simulink model "Comunicacion_taller"  (R2023a)
settings: Solver=VariableStepAuto  StartTime=0.0  StopTime=5  RelTol=1e-3
libraries: instrumentseriallib x2
settings Model: Creator=Sergio  LastModifiedBy=santi
settings DebuggingCC: UnconnectedInputMsg=warning  UnconnectedOutputMsg=warning  UnconnectedLineMsg=warning
settings ModelReferenceCC: EnableRefExpFcnMdlSchedulingChecks=on
settings RTWCC: DLArmComputeVersion=19.05

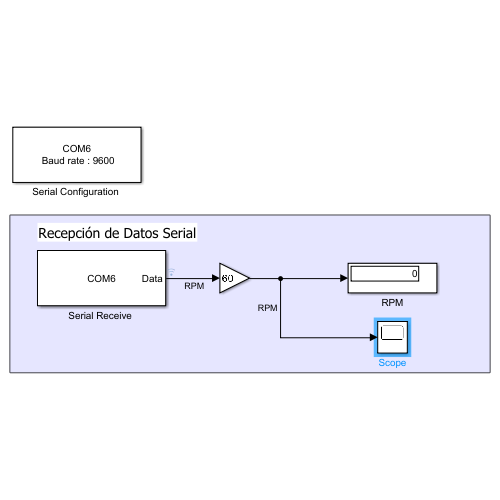
[thumbnail: Simulink's stored preview of the top-level diagram]
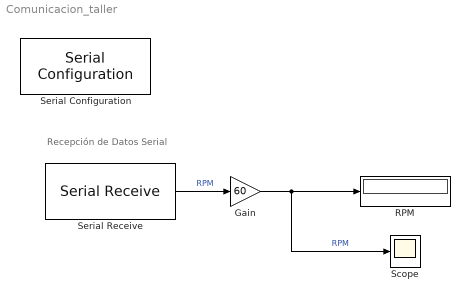
== system Comunicacion_taller ==
  note: Recepción de Datos Serial
  Gain : Gain  Gain=60
  RPM : Display
  Scope : Scope
  "Serial Configuration " : instrumentseriallib/Serial Configuration  Priority=-200000  PortSel=COM6  Port=COM6  ComPort=COM6  BaudRate=9600  DataBits=8  Parity=none  StopBits=1  ByteOrder=little-endian  FlowControl=none  Timeout=10  SimulateUsing=Interpreted execution  BlockInModel=on  aMode=1
  "Serial Receive " : instrumentseriallib/Serial Receive  Priority=1  PortSel=COM6  Port=COM6  ComPort=COM6  DataType=int8  SaveDataType=uint8  ToggleHeader=on  Header=[35]  ToggleTerminator=on  Terminator=Custom terminator  CustomTerminator=[35]  InputFormat=Column major  ToggleDataSize=on  DataSize=[1]  EnableBlockingMode=on  ActionDataUnavailable=Output last received value  ActionWhenDataUnavailable=Output last received value  CustomValue=0  SampleTime=0.05  SimulateUsing=Interpreted execution  BlockInModel=on  aMode=1
  wires:
  "Serial Receive "/1 -> Gain/1  "RPM"
  Gain/1 -> Scope/1, RPM/1  "RPM"
